simulink model "Balance_LQR"  (R2018a)
settings: Solver=FixedStepAuto  StartTime=0.0  StopTime=10.0  MaxStep=1e-2  RelTol=1e-5
PreLoadFcn:
  | modelDir = fileparts(get_param(bdroot, 'FileName'));
  | addpath(fullfile(modelDir,'../../Parameters'));
  | addpath(fullfile(modelDir,'../../Controllers/BalanceLQR'));
  | addpath(fullfile(modelDir,'../../Controllers/BalanceLQR/generated'));
  | 
  | Constants_Kugle
  | Constants_nominal
  | 
  | Parameters_Controllers
  | load('BalanceLQRgain.mat');
InitFcn:
  | Constants_Kugle
  | Constants_nominal
  | 
  | Parameters_Controllers
  | load('BalanceLQRgain.mat');
undefined symbols (not defined in the file or in its folder): BalanceLQRgain, COM_nominal, constants_nominal
settings Model: Creator=thomas  LastModifiedBy=Thomas

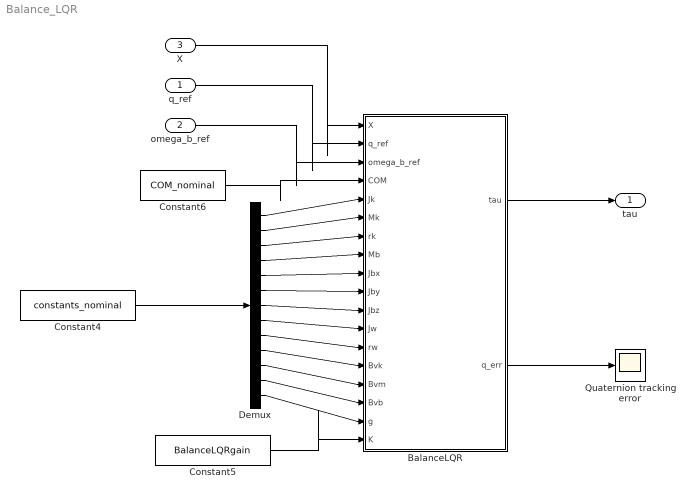
== system Balance_LQR ==
  q_ref : Inport  PortDimensions=4
  omega_b_ref : Inport  Port=2  PortDimensions=3
  X : Inport  Port=3  PortDimensions=12
  BalanceLQR : MATLAB Function  TreatAsAtomicUnit=on
  Constant4 : Constant  Value=constants_nominal
  Constant5 : Constant  Value=BalanceLQRgain
  Constant6 : Constant  Value=COM_nominal
  Demux : Demux  Outputs=13
  Quaternion tracking error : Scope
  tau : Outport
  wires:
  Constant4/1 -> Demux/1
  Constant5/1 -> BalanceLQR/18(K)
  BalanceLQR/1(tau) -> tau/1
  BalanceLQR/2(q_err) -> Quaternion tracking error/1
  Demux/1 -> BalanceLQR/5(Jk)
  Demux/2 -> BalanceLQR/6(Mk)
  Demux/3 -> BalanceLQR/7(rk)
  Demux/4 -> BalanceLQR/8(Mb)
  Demux/5 -> BalanceLQR/9(Jbx)
  Demux/6 -> BalanceLQR/10(Jby)
  Demux/7 -> BalanceLQR/11(Jbz)
  Demux/8 -> BalanceLQR/12(Jw)
  Demux/9 -> BalanceLQR/13(rw)
  Demux/10 -> BalanceLQR/14(Bvk)
  Demux/11 -> BalanceLQR/15(Bvm)
  Demux/13 -> BalanceLQR/17(g)
  Demux/12 -> BalanceLQR/16(Bvb)
  Constant6/1 -> BalanceLQR/4(COM)
  X/1 -> BalanceLQR/1(X)
  q_ref/1 -> BalanceLQR/2(q_ref)
  omega_b_ref/1 -> BalanceLQR/3(omega_b_ref)

== matlab function Balance_LQR/BalanceLQR ==
  data: X input size=12; q_ref input size=4; omega_b_ref input size=3; COM input size=3; Jk input; Mk input; rk input; Mb input; Jbx input; Jby input; Jbz input; Jw input; rw input; Bvk input; Bvm input; Bvb input; g input; K input; tau output size=3; q_err output size=4
function [tau, q_err] = BalanceLQR_(X,q_ref,omega_b_ref, COM,Jk,Mk,rk,Mb,Jbx,Jby,Jbz,Jw,rw,Bvk,Bvm,Bvb,g,  K)
    COM_X = COM(1);
    COM_Y = COM(2);
    COM_Z = COM(3);
    
    [tau, q_err] = BalanceLQR(X,q_ref,omega_b_ref,  COM_X,COM_Y,COM_Z,Jbx,Jby,Jbz,Jk,Jw,Mb,Mk,Bvb,Bvk,Bvm,rk,rw,g,  K);
end
